simulink model "KDL_act_planta_133"  (R2022b)
settings: Solver=VariableStepAuto  StartTime=0.0  StopTime=40  RelTol=1e-3
values from neighbouring files (symbols this model uses):
  FT_lat = FT_lat_function_elegante(p)    [SAS.m]
  K_DL = 1/FT_conv_balance_1gdl.Kstatic    [SAS.m]
libraries: cstblocks x1
settings Model: Creator=raulm  LastModifiedBy=raulm
settings ModelReferenceCC: EnableRefExpFcnMdlSchedulingChecks=on

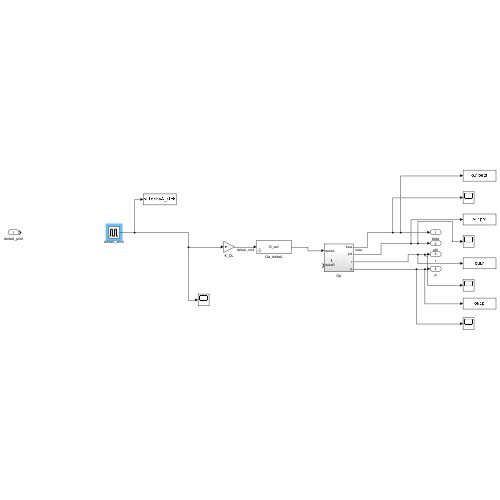
[thumbnail: Simulink's stored preview of the top-level diagram]
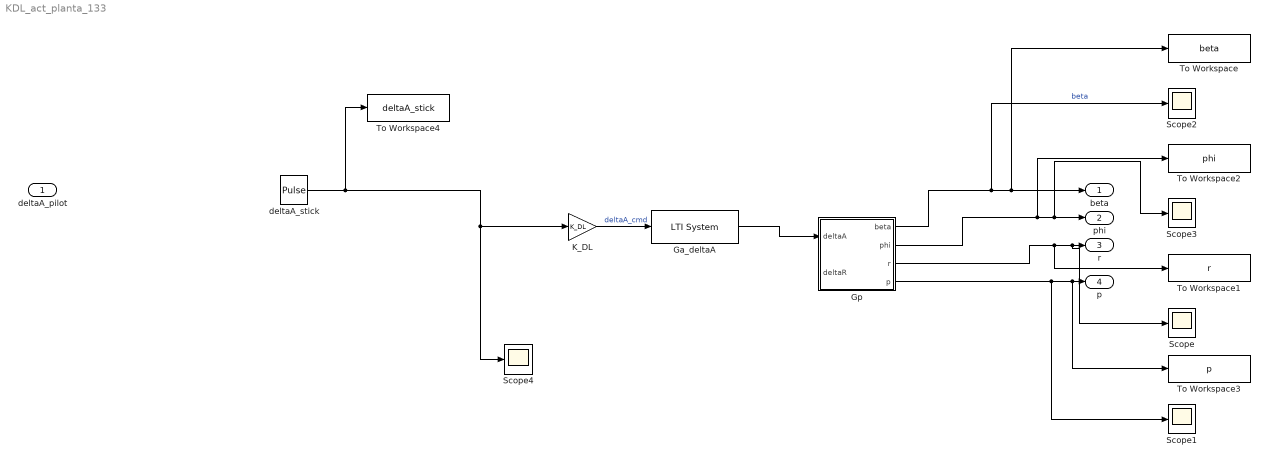
== system KDL_act_planta_133 ==
  deltaA_pilot : Inport
  Ga_deltaA : cstblocks/LTI System  sys=G_act  IC=[]
  Gp : Subsystem
  K_DL : Gain  Gain=K_DL
  Scope{,1..4} (5 alike) : Scope
  To Workspace : ToWorkspace  VariableName=beta  SampleTime=-1
      settings: Save2DSignal=2-D array (concatenate along first dimension)
  To Workspace1 : ToWorkspace  VariableName=r  SampleTime=-1
      settings: Save2DSignal=2-D array (concatenate along first dimension)
  To Workspace2 : ToWorkspace  VariableName=phi  SampleTime=-1
      settings: Save2DSignal=2-D array (concatenate along first dimension)
  To Workspace3 : ToWorkspace  VariableName=p  SampleTime=-1
      settings: Save2DSignal=2-D array (concatenate along first dimension)
  To Workspace4 : ToWorkspace  VariableName=deltaA_stick  SampleTime=-1
      settings: Save2DSignal=2-D array (concatenate along first dimension)
  deltaA_stick : DiscretePulseGenerator  PulseType=Time based  Period=100  PulseWidth=15
  beta : Outport
  phi : Outport  Port=2
  r : Outport  Port=3
  p : Outport  Port=4
  wires:
  K_DL/1 -> Ga_deltaA/1  "deltaA_cmd"
  Gp/4(p) -> Scope1/1, To Workspace3/1, p/1
  deltaA_stick/1 -> Scope4/1, K_DL/1, To Workspace4/1
  Ga_deltaA/1 -> Gp/1(deltaA)
  Gp/3(r) -> To Workspace1/1, Scope/1, r/1
  Gp/2(phi) -> To Workspace2/1, Scope3/1, phi/1
  Gp/1(beta) -> Scope2/1, To Workspace/1, beta/1  "beta"

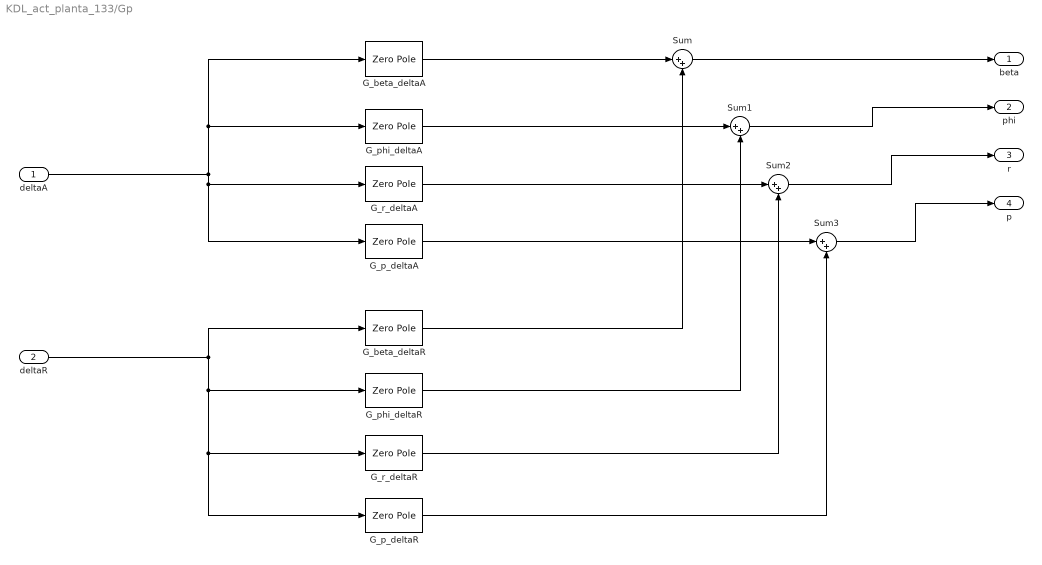
== system KDL_act_planta_133/Gp ==
  deltaA : Inport
  deltaR : Inport  Port=2
  G_beta_deltaA : ZeroPole  Zeros=FT_lat.fact.deltaA_beta.Z{1}  Poles=FT_lat.fact.deltaA_beta.P{1}  Gain=FT_lat.fact.deltaA_beta.K
  G_beta_deltaR : ZeroPole  Zeros=FT_lat.fact.deltaR_beta.Z{1}  Poles=FT_lat.fact.deltaR_beta.P{1}  Gain=FT_lat.fact.deltaR_beta.K
  G_p_deltaA : ZeroPole  Zeros=FT_lat.fact.deltaA_p.Z{1}  Poles=FT_lat.fact.deltaA_p.P{1}  Gain=FT_lat.fact.deltaA_p.K
  G_p_deltaR : ZeroPole  Zeros=FT_lat.fact.deltaR_p.Z{1}  Poles=FT_lat.fact.deltaR_p.P{1}  Gain=FT_lat.fact.deltaR_p.K
  G_phi_deltaA : ZeroPole  Zeros=FT_lat.fact.deltaA_phi.Z{1}  Poles=FT_lat.fact.deltaA_phi.P{1}  Gain=FT_lat.fact.deltaA_phi.K
  G_phi_deltaR : ZeroPole  Zeros=FT_lat.fact.deltaR_phi.Z{1}  Poles=FT_lat.fact.deltaR_phi.P{1}  Gain=FT_lat.fact.deltaR_phi.K
  G_r_deltaA : ZeroPole  Zeros=FT_lat.fact.deltaA_r.Z{1}  Poles=FT_lat.fact.deltaA_r.P{1}  Gain=FT_lat.fact.deltaA_r.K
  G_r_deltaR : ZeroPole  Zeros=FT_lat.fact.deltaR_r.Z{1}  Poles=FT_lat.fact.deltaR_r.P{1}  Gain=FT_lat.fact.deltaR_r.K
  Sum{,1..3} (4 alike) : Sum  Inputs=|++
  beta : Outport
  phi : Outport  Port=2
  r : Outport  Port=3
  p : Outport  Port=4
  wires:
  deltaR/1 -> G_p_deltaR/1, G_r_deltaR/1, G_phi_deltaR/1, G_beta_deltaR/1
  G_phi_deltaA/1 -> Sum1/1
  deltaA/1 -> G_p_deltaA/1, G_r_deltaA/1, G_phi_deltaA/1, G_beta_deltaA/1
  G_r_deltaR/1 -> Sum2/2
  G_p_deltaA/1 -> Sum3/1
  G_r_deltaA/1 -> Sum2/1
  G_beta_deltaR/1 -> Sum/2
  Sum2/1 -> r/1
  Sum3/1 -> p/1
  Sum/1 -> beta/1
  G_p_deltaR/1 -> Sum3/2
  Sum1/1 -> phi/1
  G_beta_deltaA/1 -> Sum/1
  G_phi_deltaR/1 -> Sum1/2
